simulink model "Copy_of_QP_FXP"  (R2018b)
settings: Solver=ode1  StartTime=0.0  StopTime=100  FixedStep=0.001  RelTol=1e-3
values from neighbouring files (symbols this model uses):
  kd_alpha = -100    [Para.m]
  kd_beta = 0    [Para.m]
  kd_phi = 5    [Para.m]
  ki_alpha = -1000    [Para.m]
  ki_beta = 5    [Para.m]
  ki_phi = 20    [Para.m]
  KK = lqr(A,B,Q,R)    [Para.m]
  kp_alpha = -1200    [Para.m]
  kp_beta = 80    [Para.m]
  kp_phi = 50    [Para.m]
libraries: simulink x2
settings Model: Creator=chengqian  LastModifiedBy=chengqian

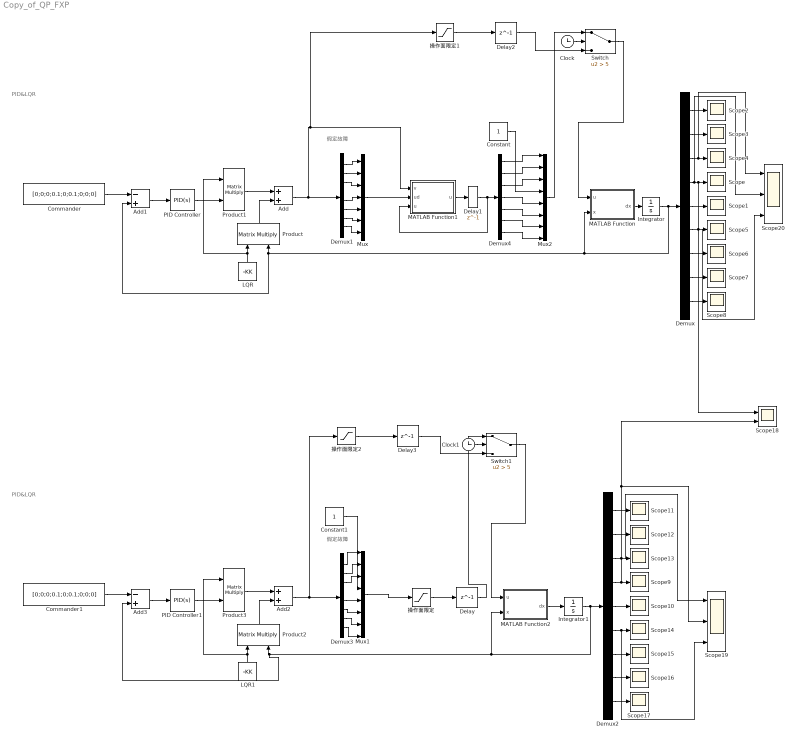
== system Copy_of_QP_FXP ==
  note: 假定故障
  note: PID&LQR
  note: 假定故障
  note: PID&LQR
  Add : Sum
  Add1 : Sum  Inputs=-+
  Add2 : Sum
  Add3 : Sum  Inputs=-+
  Clock : Clock
  Clock1 : Clock
  Commander : Constant  Value=[0;0;0;0.1;0;0.1;0;0;0]
  Commander1 : Constant  Value=[0;0;0;0.1;0;0.1;0;0;0]
  Constant : Constant
  Constant1 : Constant
  Delay : Delay  DelayLength=1  InitialCondition=[-24.88;-24.88;19.98;19.98;9.4;-9.43;-24.88;-24.88]
  Delay1 : Delay  DelayLength=1  InitialCondition=[-24.88;-24.88;19.98;9.4;-9.43;-24.88;-24.88]
  Delay2 : Delay  DelayLength=1  InitialCondition=[-24.88;-24.88;19.98;19.98;9.4;-9.43;-24.88;-24.88]
  Delay3 : Delay  DelayLength=1  InitialCondition=[-24.88;-24.88;19.98;19.98;9.4;-9.43;-24.88;-24.88]
  Demux : Demux  Outputs=9
  Demux1 : Demux  Outputs=8
  Demux2 : Demux  Outputs=9
  Demux3 : Demux  Outputs=8
  Demux4 : Demux  Outputs=7
  Integrator : Integrator  InitialCondition=[0;0;0;0;0;0;0;0;0]
  Integrator1 : Integrator  InitialCondition=[0;0;0;0;0;0;0;0;0]
  LQR : Constant  Value=-KK
  LQR1 : Constant  Value=-KK
  MATLAB Function : MATLAB Function  TreatAsAtomicUnit=on
  MATLAB Function1 : MATLAB Function  TreatAsAtomicUnit=on
  MATLAB Function2 : MATLAB Function  TreatAsAtomicUnit=on
  Mux : Mux  Inputs=7
  Mux1 : Mux  Inputs=8
  Mux2 : Mux  Inputs=8
  PID Controller : simulink/Continuous/PID Controller  Controller=PID  Form=Parallel  TimeDomain=Continuous-time  SampleTime=-1  IntegratorMethod=Forward Euler  FilterMethod=Forward Euler  ControllerParametersSource=internal  P=[0;0;kp_beta;kp_phi;0;kp_alpha;0;0;0]  I=[0;0;ki_beta;ki_phi;0;ki_alpha;0;0;0]  D=[0;0;kd_beta;kd_phi;0;kd_alpha;0;0;0]  UseFilter=on  N=1000  TunerSelectOption=Transfer Function Based (PID Tuner App)  InitialConditionSource=internal  InitialConditionForIntegrator=0  InitialConditionForFilter=0  DifferentiatorICPrevScaledInput=0  ExternalReset=none  TrackingMode=off  Kt=1  LimitOutput=off  UpperSaturationLimit=inf  LowerSaturationLimit=-inf  LinearizeAsGain=on  AntiWindupMode=none  Kb=1  POutMin=[]  POutMax=[]  IOutMin=[]  IOutMax=[]  DOutMin=[]  DOutMax=[]  NOutMin=[]  NOutMax=[]  SumOutMin=[]  SumOutMax=[]  SaturationOutMin=[]  SaturationOutMax=[]  PParamMin=[]  PParamMax=[]  IParamMin=[]  IParamMax=[]  DParamMin=[]  DParamMax=[]  NParamMin=[]  NParamMax=[]  KbParamMin=[]  KbParamMax=[]  KtParamMin=[]  KtParamMax=[]  KbOutMin=[]  KbOutMax=[]  KtOutMin=[]  KtOutMax=[]  IntegratorOutMin=[]  IntegratorOutMax=[]  FilterOutMin=[]  FilterOutMax=[]  SumI1OutMin=[]  SumI1OutMax=[]  SumI2OutMin=[]  SumI2OutMax=[]  SumI3OutMin=[]  SumI3OutMax=[]  SumI4OutMin=[]  SumI4OutMax=[]  SumDOutMin=[]  SumDOutMax=[]  DifferentiatorOutMin=[]  DifferentiatorOutMax=[]  FilterDiffOutCoefMin=[]  FilterDiffOutCoefMax=[]  ReciprocalOutMin=[]  ReciprocalOutMax=[]  SumDenOutMin=[]  SumDenOutMax=[]  SumNumOutMin=[]  SumNumOutMax=[]  DivideOutMin=[]  DivideOutMax=[]  IntegratorContinuousStateAttributes=''  IntegratorStateMustResolveToSignalObject=off  IntegratorRTWStateStorageClass=Auto  FilterContinuousStateAttributes=''  FilterStateMustResolveToSignalObject=off  FilterRTWStateStorageClass=Auto  ParallelPVariant=InternalParameters  IdealPVariant=Disabled  IVariant=InternalParameters  DVariant=InternalParameters  IntegratorVariant=Continuous  SatVariant=Disabled  AWVariant=Passthrough  PCopyVariant=Disabled  TRVariant=Disabled  FdbkBlocksVariant=Forward  IdealPFdbkVariant=Disabled  SatFdbkVariant=Disabled  DerivativeFilterVariant=ContFilter  NVariant=InternalParameters  NCopyVariant=Disabled  FilterICVariant=InternalICsFilter  IntegratorICVariant=InternalICs  ExternalResetVariant=Disabled  TRSumVariant=Passthrough  SumFdbkVariant=Disabled  SumVariant=Sum_PID
  PID Controller1 : simulink/Continuous/PID Controller  Controller=PID  Form=Parallel  TimeDomain=Continuous-time  SampleTime=-1  IntegratorMethod=Forward Euler  FilterMethod=Forward Euler  ControllerParametersSource=internal  P=[0;0;kp_beta;kp_phi;0;kp_alpha;0;0;0]  I=[0;0;ki_beta;ki_phi;0;ki_alpha;0;0;0]  D=[0;0;kd_beta;kd_phi;0;kd_alpha;0;0;0]  UseFilter=on  N=1000  TunerSelectOption=Transfer Function Based (PID Tuner App)  InitialConditionSource=internal  InitialConditionForIntegrator=0  InitialConditionForFilter=0  DifferentiatorICPrevScaledInput=0  ExternalReset=none  TrackingMode=off  Kt=1  LimitOutput=off  UpperSaturationLimit=inf  LowerSaturationLimit=-inf  LinearizeAsGain=on  AntiWindupMode=none  Kb=1  POutMin=[]  POutMax=[]  IOutMin=[]  IOutMax=[]  DOutMin=[]  DOutMax=[]  NOutMin=[]  NOutMax=[]  SumOutMin=[]  SumOutMax=[]  SaturationOutMin=[]  SaturationOutMax=[]  PParamMin=[]  PParamMax=[]  IParamMin=[]  IParamMax=[]  DParamMin=[]  DParamMax=[]  NParamMin=[]  NParamMax=[]  KbParamMin=[]  KbParamMax=[]  KtParamMin=[]  KtParamMax=[]  KbOutMin=[]  KbOutMax=[]  KtOutMin=[]  KtOutMax=[]  IntegratorOutMin=[]  IntegratorOutMax=[]  FilterOutMin=[]  FilterOutMax=[]  SumI1OutMin=[]  SumI1OutMax=[]  SumI2OutMin=[]  SumI2OutMax=[]  SumI3OutMin=[]  SumI3OutMax=[]  SumI4OutMin=[]  SumI4OutMax=[]  SumDOutMin=[]  SumDOutMax=[]  DifferentiatorOutMin=[]  DifferentiatorOutMax=[]  FilterDiffOutCoefMin=[]  FilterDiffOutCoefMax=[]  ReciprocalOutMin=[]  ReciprocalOutMax=[]  SumDenOutMin=[]  SumDenOutMax=[]  SumNumOutMin=[]  SumNumOutMax=[]  DivideOutMin=[]  DivideOutMax=[]  IntegratorContinuousStateAttributes=''  IntegratorStateMustResolveToSignalObject=off  IntegratorRTWStateStorageClass=Auto  FilterContinuousStateAttributes=''  FilterStateMustResolveToSignalObject=off  FilterRTWStateStorageClass=Auto  ParallelPVariant=InternalParameters  IdealPVariant=Disabled  IVariant=InternalParameters  DVariant=InternalParameters  IntegratorVariant=Continuous  SatVariant=Disabled  AWVariant=Passthrough  PCopyVariant=Disabled  TRVariant=Disabled  FdbkBlocksVariant=Forward  IdealPFdbkVariant=Disabled  SatFdbkVariant=Disabled  DerivativeFilterVariant=ContFilter  NVariant=InternalParameters  NCopyVariant=Disabled  FilterICVariant=InternalICsFilter  IntegratorICVariant=InternalICs  ExternalResetVariant=Disabled  TRSumVariant=Passthrough  SumFdbkVariant=Disabled  SumVariant=Sum_PID
  Product{,1..3} (4 alike) : Product  Multiplication=Matrix(*)
  Scope{,1..17} (18 alike) : Scope
  Scope18 : Scope  NumInputPorts=2
  Scope19 : Scope  NumInputPorts=3
  Scope20 : Scope  NumInputPorts=3
  Switch : Switch  Criteria=u2 > Threshold  Threshold=5
  Switch1 : Switch  Criteria=u2 > Threshold  Threshold=5
  操作面限定 : Saturate  UpperLimit=[25;25;26;26;30;30;30;30]  LowerLimit=-[25;25;15;15;60;60;30;30]
  操作面限定1 : Saturate  UpperLimit=[25;25;26;26;30;30;30;30]  LowerLimit=-[25;25;15;15;60;60;30;30]
  操作面限定2 : Saturate  UpperLimit=[25;25;26;26;30;30;30;30]  LowerLimit=-[25;25;15;15;60;60;30;30]
  wires:
  MATLAB Function/1(dx) -> Integrator/1
  LQR/1 -> Product1/1, Product/1
  Integrator/1 -> Demux/1, Add1/2, Product/2, MATLAB Function/2(x)
  Product/1 -> Add/2
  PID Controller/1 -> Product1/2
  Add1/1 -> PID Controller/1
  Commander/1 -> Add1/1
  Product1/1 -> Add/1
  Add/1 -> 操作面限定1/1, MATLAB Function1/1(v), Demux1/1
  Demux/5 -> Scope1/1
  Demux1/1 -> Mux/1
  Demux1/5 -> Mux/4
  Demux1/6 -> Mux/5
  Demux1/7 -> Mux/6
  Demux/1 -> Scope2/1
  Demux/2 -> Scope3/1
  Demux/3 -> Scope20/1, Scope4/1
  Demux/6 -> Scope20/3, Scope5/1
  Demux/9 -> Scope8/1
  Demux/8 -> Scope7/1
  Demux/7 -> Scope6/1
  MATLAB Function1/1(u) -> Delay1/1
  Mux/1 -> MATLAB Function1/2(ud)
  Demux1/8 -> Mux/7
  Delay1/1 -> Demux4/1, MATLAB Function1/3("u ")
  LQR1/1 -> Product3/1, Product2/1
  Demux3/8 -> Mux1/8
  Demux3/6 -> Mux1/6
  Demux3/7 -> Mux1/7
  Demux3/5 -> Mux1/5
  Demux2/2 -> Scope12/1
  Demux2/1 -> Scope11/1
  Demux2/8 -> Scope16/1
  Demux2/5 -> Scope10/1
  PID Controller1/1 -> Product3/2
  Product3/1 -> Add2/1
  Commander1/1 -> Add3/1
  Add3/1 -> PID Controller1/1
  Demux2/6 -> Scope19/3, Scope14/1
  MATLAB Function2/1(dx) -> Integrator1/1
  Demux2/3 -> Scope19/1, Scope13/1
  Demux2/9 -> Scope17/1
  Demux2/7 -> Scope15/1
  Product2/1 -> Add2/2
  Demux2/4 -> Scope19/2, Scope18/2, Scope9/1
  Mux1/1 -> 操作面限定/1
  Demux3/1 -> Mux1/1
  Demux4/1 -> Mux2/1
  Demux4/5 -> Mux2/6
  Demux4/6 -> Mux2/7
  Demux4/7 -> Mux2/8
  操作面限定/1 -> Delay/1
  Clock/1 -> Switch/2
  操作面限定1/1 -> Delay2/1
  Mux2/1 -> Switch/1
  Delay2/1 -> Switch/3
  Delay3/1 -> Switch1/3
  操作面限定2/1 -> Delay3/1
  Add2/1 -> 操作面限定2/1, Demux3/1
  Clock1/1 -> Switch1/2
  Delay/1 -> Switch1/1
  Demux1/3 -> Mux/3
  Integrator1/1 -> Demux2/1, Add3/2, Product2/2, MATLAB Function2/2(x)
  Switch/1 -> MATLAB Function/1(u)
  Switch1/1 -> MATLAB Function2/1(u)
  Demux1/2 -> Mux/2
  Demux3/3 -> Mux1/3
  Demux4/2 -> Mux2/2
  Demux4/3 -> Mux2/3
  Constant/1 -> Mux2/4
  Demux4/4 -> Mux2/5
  Demux3/2 -> Mux1/2
  Constant1/1 -> Mux1/4
  Demux/4 -> Scope18/1, Scope/1, Scope20/2

== matlab function Copy_of_QP_FXP/MATLAB Function1 ==
  data: v input; ud input; u output; u input size=7
function u  = my_fxp_alloc(v,ud,u)

% FXP_ALLOC - Control allocation using a fixed-point iterations.
%
%  [u,iter] = fxp_alloc(B,v,umin,umax,[Wv,Wu,ud,gamma,u0,imax])
%
% Solves the weighted, bounded least-squares problem
% 
%   min ||Wu(u-ud)||^2 + gamma ||Wv(Bu-v)||^2
%
%   subj. to  umin <= u <= umax
% 
% using a fixed-point iteration algorithm.
%
%  Inputs:
%  -------
% B     control effectiveness matrix (k x m)
%%假设去掉第三个
B = 0.08*eye(8,7);
umin = -[25;25;15;60;60;30;30];
umax = [25;25;26;30;30;30;30];
% v     commanded virtual control (k x 1)
% umin  lower position limits (m x 1)
% umax  upper position limits (m x 1)
% Wv    virtual control weighting matrix (k x k) [I]
Wv = eye(8);
Wu = eye(7);
gam = 1/0.0005;
% Wu    control weighting matrix (m x m) [I]
% ud    desired control (m x 1) [0]
% gamma weight (scalar) [1e3]
% u0    initial point (m x 1)
u0 = [-24.88;-24.88;19.98;9.4;-9.43;-24.88;-24.88];
% imax  no. of iterations [100]
imax = 100;
% 
%  Outputs:
%  -------
% u     (approximately) optimal solution
% iter  no. of iterations
%
% See also: WLS_ALLOC, WLSC_ALLOC, IP_ALLOC, QP_SIM.
  
% Number of variables
  m = 7;
  
  % Set default values of optional arguments
%   if nargin < 10
%     imax = 100; % Heuristic value
%     [k,m] = size(B);
%     if nargin < 9, u = (umin+umax)/2; end
%     if nargin < 8, gam = 1e3;         end
%     if nargin < 7, ud = zeros(m,1);  end
%     if nargin < 6, Wu = eye(m);      end
%     if nargin < 5, Wv = eye(k);      end
%   end

  % Change of variables.
  x = u - ud;
  xmin = umin - ud;
  xmax = umax - ud;
  
  % Compute the weight epsilon used by Burken et al.
  e = 1/(gam+1);
  
  % m = number of variables (actuators)
  %m = size(B,2);
  
  % Notational differences: Q1 = Wu'Wu
  %			    Q2 = Wv'Wv
  %			    CzBu*-dz = v
  
  % Common factor.
  BzT_Q1 = B'*Wv'*Wv;
  % Just above eq. (25).
  H = (1-e) * (BzT_Q1 * B) + e*Wu'*Wu;
  % Eq. (25).
  w = 1/norm(H,'fro');
  % Matrices used for updating solution: 
  % u[k] = sat(Fv-Gu[k-1])
  Fv = (1-e) * w * BzT_Q1 * v;
  G  = w*H - eye(m);
    
  for iter = 1:imax
    % Compute next point without considering the constraints.
    x = Fv - G*x;
    % Saturate to box constraints.
    x = max(xmin,min(xmax,x));
  end
    
  % Back to original variables.
  u = x + ud;

== matlab function Copy_of_QP_FXP/MATLAB Function ==
  data: u input size=8; dx output size=9; x input
function dx = fcn(u,x)

%%x = [p;r;beta;phi;psi;alpha;q;theta;v].
%%u = [delta_rei;delta_lei;delta_rfl;delta_lfl;delta_rvr;delta_lvr;delta_reo;delta_leo]

Alat = [-0.099170  0.020570  2.805001  0.000001 0.000001;
        -0.002640 -0.031920 -0.674200  0        0;
        -0.108500 -0.994000 -0.029750  0.010210 0.000034;
         1.0       0.016090 -0.000148  0.000016 0;
         0         1.0       0.000120 -0.000013 0.000122];
Alon = [-0.064190   1.000001 0.000844 -0.000130;
        -1.424000  -0.051730 0.000001  0;
        -0.0000138  1.0      0.000014  0.000003;
        -0.550041   0       -0.559090 -0.013375];

A = [Alat zeros(5,4);
     zeros(4,5) Alon];
B = [-0.2883  0.2883 -0.8654  0.8654 -0.0000  0.0025 -0.2883  0.2883;
     -0.0959  0.0959  0.2079 -0.2079 -0.0045 -0.0051 -0.0959  0.0959;
      0.0000  0.0000  0.0003 -0.0003 -0.0001  0       0       0;
      0       0       0       0       0       0       0       0;
      0       0       0       0       0       0       0       0;
     -0.0005 -0.0005 -0.0019 -0.0019 -0.0005  0.0004 -0.0005 -0.0005;
     -0.0857 -0.0857 -0.5263 -0.5263  0.0098 -0.0073 -0.0857 -0.0857;
      0       0       0       0       0       0       0       0;
     -0.0034 -0.0034 -0.1285 -0.1285  0.0011 -0.0011 -0.0041 -0.0041]; 
dx = A*x + B*u;

== matlab function Copy_of_QP_FXP/MATLAB Function2 ==
  data: u input size=8; dx output size=9; x input
function dx = fcn(u,x)

%%x = [p;r;beta;phi;psi;alpha;q;theta;v].
%%u = [delta_rei;delta_lei;delta_rfl;delta_lfl;delta_rvr;delta_lvr;delta_reo;delta_leo]

Alat = [-0.099170  0.020570  2.805001  0.000001 0.000001;
        -0.002640 -0.031920 -0.674200  0        0;
        -0.108500 -0.994000 -0.029750  0.010210 0.000034;
         1.0       0.016090 -0.000148  0.000016 0;
         0         1.0       0.000120 -0.000013 0.000122];
Alon = [-0.064190   1.000001 0.000844 -0.000130;
        -1.424000  -0.051730 0.000001  0;
        -0.0000138  1.0      0.000014  0.000003;
        -0.550041   0       -0.559090 -0.013375];

A = [Alat zeros(5,4);
     zeros(4,5) Alon];
B = [-0.2883  0.2883 -0.8654  0.8654 -0.0000  0.0025 -0.2883  0.2883;
     -0.0959  0.0959  0.2079 -0.2079 -0.0045 -0.0051 -0.0959  0.0959;
      0.0000  0.0000  0.0003 -0.0003 -0.0001  0       0       0;
      0       0       0       0       0       0       0       0;
      0       0       0       0       0       0       0       0;
     -0.0005 -0.0005 -0.0019 -0.0019 -0.0005  0.0004 -0.0005 -0.0005;
     -0.0857 -0.0857 -0.5263 -0.5263  0.0098 -0.0073 -0.0857 -0.0857;
      0       0       0       0       0       0       0       0;
     -0.0034 -0.0034 -0.1285 -0.1285  0.0011 -0.0011 -0.0041 -0.0041]; 
 Bz = [-0.2883  0.2883 -0.8654   -0.0000  0.0025 -0.2883  0.2883;
     -0.0959  0.0959  0.2079  -0.0045 -0.0051 -0.0959  0.0959;
      0.0000  0.0000  0.0003  -0.0001  0       0       0;
      0       0       0              0       0       0       0;
      0       0       0              0       0       0       0;
     -0.0005 -0.0005 -0.0019  -0.0005  0.0004 -0.0005 -0.0005;
     -0.0857 -0.0857 -0.5263   0.0098 -0.0073 -0.0857 -0.0857;
      0       0       0              0       0       0       0;
     -0.0034 -0.0034 -0.1285   0.0011 -0.0011 -0.0041 -0.0041];

dx = A*x + B*u;
